simulink model "rb_system"  (R2024b)
settings: Solver=VariableStepAuto  StartTime=0.0  StopTime=10.0  RelTol=1e-3
undefined symbols (not defined in the file or in its folder): cf, de0, de1, de2, ke, ks, M, num0, num1, rg
settings Model: Creator=hoang  LastModifiedBy=hoang

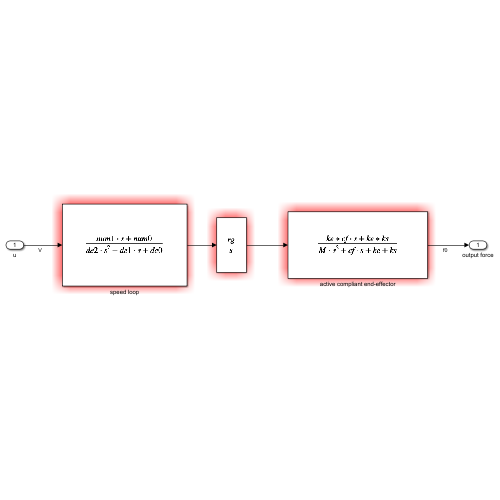
[thumbnail: Simulink's stored preview of the top-level diagram]
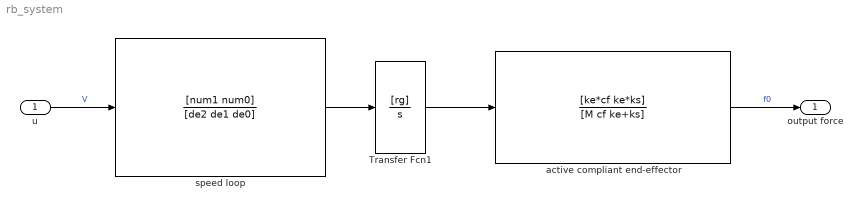
== system rb_system ==
  u : Inport
  Transfer Fcn1 : TransferFcn  Numerator=[rg]  Denominator=[1 0]
  active compliant end-effector : TransferFcn  Numerator=[ke*cf ke*ks]  Denominator=[M cf ke+ks]
  speed loop : TransferFcn  Numerator=[num1 num0]  Denominator=[de2 de1 de0]
  output force : Outport  VectorParamsAs1DForOutWhenUnconnected=off
  wires:
  speed loop/1 -> Transfer Fcn1/1
  u/1 -> speed loop/1  "V"
  Transfer Fcn1/1 -> active compliant end-effector/1
  active compliant end-effector/1 -> output force/1  "f0"
